simulink model "watertank"  (R2021b)
settings: Solver=FixedStepAuto  StartTime=0.0  StopTime=inf  FixedStep=0.1  RelTol=1e-3
StopFcn:
  | if isLogging
  |     outputJson = jsonencode(struct("simTime", output.simTime, "percentFull", simOutput.percentFull, "pump", simInput.pump, "valve", simInput.valve));
  |     fprintf(outputFile, "%s]", outputJson);
  |     fclose(outputFile);
  | end
model workspace (MAT data in the model file):
  Obj = Simulink.NumericType
  Obj.DataTypeMode = 'Double'
  Obj.SignednessBool = 1
  Obj.WordLength = 64
  Obj.FixedExponent = 0
  Obj.SlopeAdjustmentFactor = 1
  Obj.Bias = 0
  Obj.DataTypeOverride = 'Inherit'
  Obj.IsAlias = 0
  Obj.DataScope = 'Auto'
  PLC_IP_Address = 'localhost'
  pump = 1
  valve = 1
values from neighbouring files (symbols this model uses):
  simInput = struct("pump", 1, "valve", 1)    [initModel.m]
libraries: sh_lib x9, nesl_utility x7, fl_lib x4
PauseFcn:
  | if exist("fixedStepSize", "var") == 0
  |     fixedStepSize = simOutput.SimulationMetadata.ModelInfo.SolverInfo.FixedStepSize;
  | end
  | output.simTime = simOutput.SimulationMetadata.ModelInfo.StopTime - fixedStepSize;
  | output.percentFull = simOutput.percentFull;
ContinueFcn:
  | if isLogging
  |     outputJson = jsonencode(struct("simTime", output.simTime, "percentFull", simOutput.percentFull, "pump", simInput.pump, "valve", simInput.valve));
  |     fprintf(outputFile, "%s,", outputJson);
  | end
settings Model: PacingRate=0.600000  Creator=CCRE  LastModifiedBy=fastsim
settings SolverCC: AlgebraicLoopSolver=TrustRegion
settings DataIOCC: SaveOutput=off  SignalLogging=off  DSMLogging=off  SaveTime=off  ReturnWorkspaceOutputsName=simOutput
settings DebuggingCC: SFMachineParentedDataDiag=warning  ArithmeticOperatorsInVariantConditions=warning
settings SFSimCC: SimUseLocalCustomCode=off  CustomCodeUndefinedFunction=UseInterfaceOnly
settings RTWCC: GenerateReport=on  RTWUseLocalCustomCode=off  BuildConfiguration=Faster Runs  LaunchReport=on
settings CodeAppCC: StateflowObjectComments=on
settings SimscapeCC: SimscapeNormalizeSystem=off

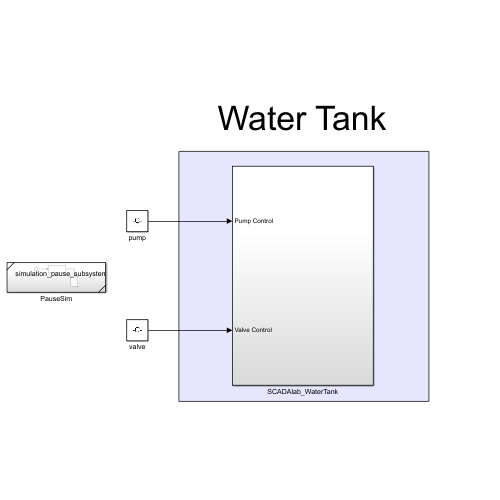
[thumbnail: Simulink's stored preview of the top-level diagram]
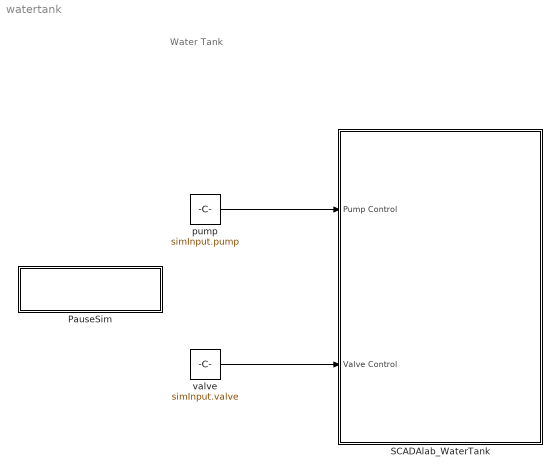
== system watertank ==
  note: Water Tank
  PauseSim : Subsystem  ReferencedSubsystem=simulation_pause_subsystem
  SCADAlab_WaterTank : Subsystem
  pump : Constant  Value=simInput.pump
  valve : Constant  Value=simInput.valve
  wires:
  pump/1 -> SCADAlab_WaterTank/1(Pump Control)
  valve/1 -> SCADAlab_WaterTank/2("Valve Control ")

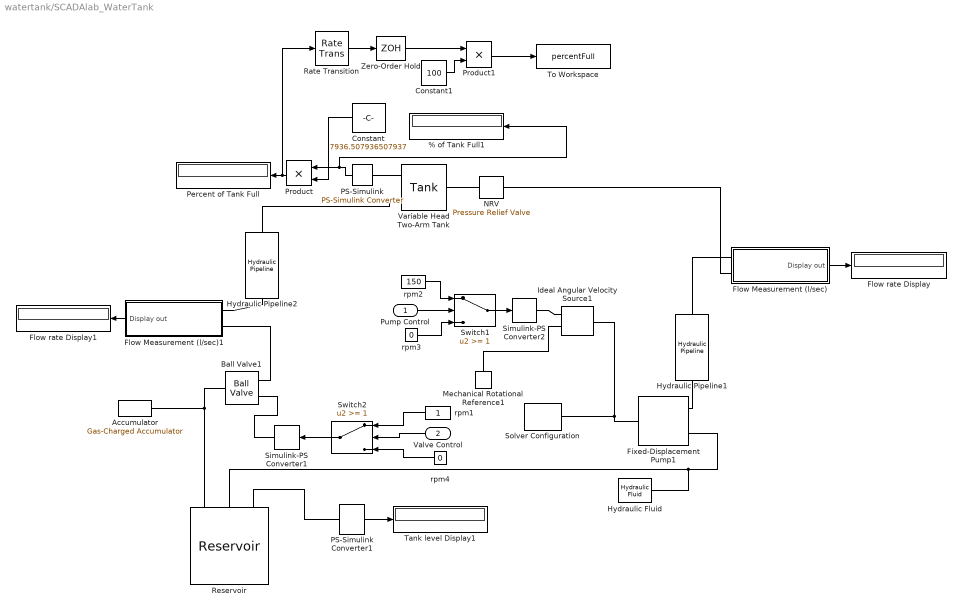
== system watertank/SCADAlab_WaterTank ==
  Pump Control : Inport
  "Valve Control " : Inport  Port=2
  % of Tank Full1 : Display
  Accumulator : sh_lib/Accumulators/Gas-Charged Accumulator  capacity=20 gal  dead_volume=10 gal  pr_preload=0 Pa  k_sh=1.4  stiff_coeff=1e5 Pa/m^3  penetr_coeff=1e5 s*Pa/m^6  flow_rate_specify=off  flow_rate_priority=None  flow_rate=0.005 m^3/s  flow_rate_nominal_specify=off  flow_rate_nominal_unit=m^3/s  flow_rate_nominal_value=1  liquid_volume_specify=on  liquid_volume_priority=High  liquid_volume=0 m^3  liquid_volume_nominal_specify=off  liquid_volume_nominal_unit=m^3  liquid_volume_nominal_value=1  liquid_pressure_specify=off  liquid_pressure_priority=None  liquid_pressure=1.01325e+5 Pa  liquid_pressure_nominal_specify=off  liquid_pressure_nominal_unit=Pa  liquid_pressure_nominal_value=1
      settings: SourceProductBaseCode=SH  InternalSimscapePortConfiguration="{\"Bottom\":[],\"Left\":[],\"Right\":[{\"id\":\"A\",\"label\":\"A\",\"type\":\"foundation.hydraulic.hydraulic\"}],\"Top\":[]}"
  Ball Valve1 : sh_lib/Valves/Flow Control Valves/Ball Valve  valve_seat_spec=1  cone_ang=120 deg  d_ball=3.2 cm  d_orif=3 cm  x_0=0 cm  C_d=0.65  A_leak=1e-12 m^2  lam_spec=2  B_lam=0.999  Re_cr=10  flow_rate_specify=off  flow_rate_priority=None  flow_rate=0.001 m^3/s  flow_rate_nominal_specify=off  flow_rate_nominal_unit=m^3/s  flow_rate_nominal_value=1  pressure_drop_specify=off  pressure_drop_priority=None  pressure_drop=0 Pa  pressure_drop_nominal_specify=off  pressure_drop_nominal_unit=Pa  pressure_drop_nominal_value=1
      settings: SourceProductBaseCode=SH  InternalSimscapePortConfiguration="{\"Bottom\":[],\"Left\":[{\"id\":\"S\",\"label\":\"S\",\"type\":\"input\"},{\"id\":\"A\",\"label\":\"A\",\"type\":\"foundation.hydraulic.hydraulic\"}],\"Right\":[{\"id\":\"B\",\"label\":\"B\",\"type\":\"foundation.hydraulic.hydraulic\"}],\"Top\":[]}"
  Constant : Constant  Value=7936.507936507937
  Constant1 : Constant  Value=100
  Fixed-Displacement Pump1 : sh_lib/Pumps and Motors/Fixed-Displacement Pump  D=0.0271551724137931 l/rev  loss_spec=1  w_nominal=3600 rpm  pr_nominal=.9 bar  visc_nominal=18 cSt  dens_nominal=980 kg/m^3  efficiency_vol=0.92  no_load_torque=0 N*m  torque_pressure_coeff=0.15915*(.0000001)*((0.92)/(0.8)-1 ) N*m/Pa  p_diff_eff_TLU=[100000.0, 1000000.0, 2000000.0] Pa  omega_eff_TLU=[25.0, 50.0, 100.0, 200.0, 300.0, 400.0] rad/s  vol_eff_TLU=[0.816, 0.908, 0.954, 0.977, 0.981, 0.984; 0.325, 0.663, 0.831, 0.916, 0.925, 0.946; 0.137, 0.568, 0.78, 0.892, 0.893, 0.91]  mech_eff_TLU=[0.996, 0.996, 0.996, 0.996, 0.996, 0.996; 0.988, 0.989, 0.989, 0.989, 0.989, 0.99; 0.981, 0.981, 0.982, 0.982, 0.983, 0.984]  p_diff_loss_TLU=[100000.0, 1000000.0, 2000000.0] Pa  omega_loss_TLU=[25.0, 50.0, 100.0, 200.0, 300.0, 400.0] rad/s  vol_loss_TLU=[0.023, 0.023, 0.023, 0.023, 0.0285, 0.032; 0.0844, 0.0842, 0.0845, 0.084, 0.1125, 0.108; 0.1079, 0.108, 0.11, 0.108, 0.1605, 0.18] * 1e-3 m^3/s  mech_loss_TLU=[0.002, 0.002, 0.002, 0.002, 0.002, 0.002; 0.0607, 0.0556, 0.0556, 0.0556, 0.0556, 0.0505; 0.1937, 0.1937, 0.1833, 0.1833, 0.1729, 0.1626] N*m  pressure_threshold=1e5 Pa  omega_threshold=10 rad/s  quadrant_check=0  pressure_check=0  min_valid_pressure=0 Pa  vol_eff_min=1e-3  vol_eff_max=1  mech_eff_min=1e-3  mech_eff_max=1
      settings: SourceProductBaseCode=SH  InternalSimscapePortConfiguration="{\"Bottom\":[],\"Left\":[{\"id\":\"S\",\"label\":\"S\",\"type\":\"foundation.mechanical.rotational.rotational\"}],\"Right\":[{\"id\":\"P\",\"label\":\"P\",\"type\":\"foundation.hydraulic.hydraulic\"},{\"id\":\"T\",\"label\":\"T\",\"type\":\"foundation.hydraulic.hydraulic\"}],\"Top\":[]}"
  Flow Measurement (l/sec) : Subsystem
  Flow Measurement (l/sec)1 : Subsystem
  Flow rate Display : Display
  Flow rate Display1 : Display
  Hydraulic Fluid : sh_lib/Hydraulic Utilities/Hydraulic Fluid  DataSource=1  SelFluid=24  SysTemp=30  TrapAir=0.005  ViscDerFactor=1  range_error=1
  Hydraulic Pipeline1 : sh_lib/Pipelines/Hydraulic Pipeline  cs_type=1  d_in=.5 cm  area=1e-4 m^2  D_h=0.0112 m  s_factor=64  length=140 cm  length_ad=140 cm  roughness=1.5e-2 cm  Re_lam=2e+3  Re_turb=4e+3  wall_type=1  pr_r_coef=2e-12 m/Pa  time_const=0.01 s  k_sh=1.4  initial_pressure=0 Pa
      settings: SourceProductBaseCode=SH  InternalSimscapePortConfiguration="{\"Bottom\":[],\"Left\":[{\"id\":\"A\",\"label\":\"A\",\"type\":\"foundation.hydraulic.hydraulic\"}],\"Right\":[{\"id\":\"B\",\"label\":\"B\",\"type\":\"foundation.hydraulic.hydraulic\"}],\"Top\":[]}"
  Hydraulic Pipeline2 : sh_lib/Pipelines/Hydraulic Pipeline  cs_type=1  d_in=.7 cm  area=1e-4 m^2  D_h=0.0112 m  s_factor=64  length=90 cm  length_ad=10 cm  roughness=1.5e-3 cm  Re_lam=2e+3  Re_turb=4e+3  wall_type=1  pr_r_coef=2e-12 m/Pa  time_const=0.01 s  k_sh=1.4  initial_pressure=0 Pa
      settings: SourceProductBaseCode=SH  InternalSimscapePortConfiguration="{\"Bottom\":[],\"Left\":[{\"id\":\"A\",\"label\":\"A\",\"type\":\"foundation.hydraulic.hydraulic\"}],\"Right\":[{\"id\":\"B\",\"label\":\"B\",\"type\":\"foundation.hydraulic.hydraulic\"}],\"Top\":[]}"
  Ideal Angular Velocity Source1 : fl_lib/Mechanical/Mechanical Sources/Ideal Angular Velocity Source
  Mechanical Rotational Reference1 : fl_lib/Mechanical/Rotational Elements/Mechanical Rotational Reference
  NRV : sh_lib/Valves/Pressure Control Valves/Pressure Relief Valve  valve_area_spec=1  p_diff_TLU=[30.15e5 : 15e3 : 31.35e5] Pa  area_TLU=[1 : 1 : 9] .* 1e-5 m^2  area_max=1e-4 m^2  pres_set=0.001 Pa  reg_range=5e5 Pa  C_d=0.7  A_leak=1e-12 m^2  lam_spec=2  B_lam=0.999  Re_cr=12  dynamic=0  tau=0.1 s  area_init=1e-12 m^2
      settings: SourceProductBaseCode=SH  InternalSimscapePortConfiguration="{\"Bottom\":[],\"Left\":[{\"id\":\"A\",\"label\":\"A\",\"type\":\"foundation.hydraulic.hydraulic\"}],\"Right\":[{\"id\":\"B\",\"label\":\"B\",\"type\":\"foundation.hydraulic.hydraulic\"}],\"Top\":[]}"
  "PS-Simulink " : nesl_utility/PS-Simulink Converter  PhysicalDomain=network_engine_domain  SubClassName=ps_output  LeftPortType=input  RightPortType=output  PseudoPeriodic=off  Frequencies=[]  Unit=1  AffineConversion=off
      settings: SourceProductBaseCode=PW,SS
  PS-Simulink Converter1 : nesl_utility/PS-Simulink Converter  PhysicalDomain=network_engine_domain  SubClassName=ps_output  LeftPortType=input  RightPortType=output  PseudoPeriodic=off  Frequencies=[]  Unit=1  AffineConversion=off
      settings: SourceProductBaseCode=PW,SS
  Percent of Tank Full : Display
  Product : Product
  Product1 : Product
  Rate Transition : RateTransition
  Reservoir : sh_lib/Hydraulic Utilities/Reservoir  press=0 Pa  init_volume=1000000 l  ret_diam=.5 cm  loss_coeff=1
      settings: SourceProductBaseCode=SH  InternalSimscapePortConfiguration="{\"Bottom\":[],\"Left\":[{\"id\":\"V\",\"label\":\"V\",\"type\":\"output\"},{\"id\":\"P\",\"label\":\"P\",\"type\":\"foundation.hydraulic.hydraulic\"},{\"id\":\"R\",\"label\":\"R\",\"type\":\"foundation.hydraulic.hydraulic\"}],\"Right\":[],\"Top\":[]}"
  Simulink-PS Converter1 : nesl_utility/Simulink-PS Converter  PhysicalDomain=network_engine_domain  SubClassName=ps_input  LeftPortType=input  RightPortType=output  PseudoPeriodic=off  Frequencies=[]  NoiseDistribution=none  NoiseParameters=[]  Unit=1  AffineConversion=off  FilteringAndDerivatives=zero  SimscapeFilterOrder=1  InputFilterTimeConstant=0.001  UdotUserProvided=1
      settings: SourceProductBaseCode=PW,SS
  Simulink-PS Converter2 : nesl_utility/Simulink-PS Converter  PhysicalDomain=network_engine_domain  SubClassName=ps_input  LeftPortType=input  RightPortType=output  PseudoPeriodic=off  Frequencies=[]  NoiseDistribution=none  NoiseParameters=[]  Unit=1  AffineConversion=off  FilteringAndDerivatives=zero  SimscapeFilterOrder=1  InputFilterTimeConstant=0.001  UdotUserProvided=1
      settings: SourceProductBaseCode=PW,SS
  Solver Configuration : nesl_utility/Solver Configuration  PhysicalDomain=network_engine_domain  SubClassName=solver  LeftPortType=input  RightPortType=generic  Tones=[]  Harmonics=[]  SimulateNoise=off  Profile=off  UseLocalSampling=off  EnableSwitchedLinearOptims=on  FrequencyDomain=off  UseCCode=off  RelTol=0.001  AbsTol=1e-06  MinStep=1e-09  ToWorkspace=off  RevertToSquareIcSolve=off  NumHomotopyIterations=100  PhasorMode=off  PhasorModeNumHarmonics=1  DoDC=off  ResidualTolerance=1  UseLocalSolver=on  LocalSolverChoice=NE_TRAPEZOIDAL_ADVANCER  LocalSolverSampleTime=0.1  DoFixedCost=on  MaxNonlinIter=12  MaxModeIter=2  ComputeImpulses=off  ImpulseIterations=2  LinearAlgebra=Full  EquationFormulation=NE_TIME_EF  DelaysMemoryBudget=1024  AutomaticFiltering=on  FilteringTimeConstant=0.001  PartitionStorageMethod=AS_NEEDED  PartitionMemoryBudget=1024  PartitionMethod=FAST
      settings: SourceProductBaseCode=PW,SS
  Switch1 : Switch  Threshold=1
  Switch2 : Switch  Threshold=1
  Tank level Display1 : Display
  To Workspace : ToWorkspace  VariableName=percentFull  SampleTime=-1
      settings: MaxDataPoints=1  Save2DSignal=2-D array (concatenate along first dimension)
  Variable Head Two-Arm Tank : sh_lib/Low-Pressure Blocks/Tank  press=0 Pa  level_spec=1  tank_area=.0314 m^2  fluid_volume_tab=[ 0 0.0028 0.0065 0.0114 0.0176 0.0252 0.0344 0.0436 0.0512 0.0574 0.0623 0.066 0.0688 0.0707 0.07199999999999999 0.0727 ] m^3  fluid_level_tab=[ 0 0.02 0.04 0.06 0.08 0.1 0.12 0.14 0.16 0.18 0.2 0.22 0.24 0.26 0.28 0.3 ] m  interp_method=1  extrap_method=1  pipe_diam=0.02 m  loss_coeff=1.2  g=9.80665 m/s^2  min_level=1e-3 m  fluid_level_check=0  volume_specify=on  volume_priority=High  volume=0 l  volume_nominal_specify=off  volume_nominal_unit=l  volume_nominal_value=1  level_specify=off  level_priority=None  level=0.025 m  level_nominal_specify=off  level_nominal_unit=m  level_nominal_value=1  pipe_diam_A=0.2 m  loss_coeff_A=1.2  height_B=38 cm  pipe_diam_B=0.2 m  loss_coeff_B=1.2  height_C=0.8 m  pipe_diam_C=0.02 m  loss_coeff_C=1.2
      settings: SourceProductBaseCode=SH  InternalSimscapePortConfiguration="{\"Bottom\":[],\"Left\":[{\"id\":\"B\",\"label\":\"B\",\"type\":\"foundation.hydraulic.hydraulic\"}],\"Right\":[{\"id\":\"V\",\"label\":\"V\",\"type\":\"output\"},{\"id\":\"A\",\"label\":\"A\",\"type\":\"foundation.hydraulic.hydraulic\"}],\"Top\":[]}"
  Zero-Order Hold : ZeroOrderHold  SampleTime=0.1
  rpm1 : Constant
  rpm2 : Constant  Value=150
  rpm3 : Constant  Value=0
  rpm4 : Constant  Value=0
  wires:
  Flow Measurement (l/sec)1/1(Display out) -> Flow rate Display1/1
  PS-Simulink Converter1/1 -> Tank level Display1/1
  Flow Measurement (l/sec)/1(Display out) -> Flow rate Display/1
  Constant/1 -> Product/2
  "PS-Simulink "/1 -> % of Tank Full1/1, Product/1
  rpm3/1 -> Switch1/3
  rpm2/1 -> Switch1/1
  Pump Control/1 -> Switch1/2
  Switch1/1 -> Simulink-PS Converter2/1
  rpm4/1 -> Switch2/3
  rpm1/1 -> Switch2/1
  Switch2/1 -> Simulink-PS Converter1/1
  "Valve Control "/1 -> Switch2/2
  Product/1 -> Rate Transition/1, Percent of Tank Full/1
  Rate Transition/1 -> Zero-Order Hold/1
  Constant1/1 -> Product1/2
  Zero-Order Hold/1 -> Product1/1
  Product1/1 -> To Workspace/1
  connections:
  Variable Head Two-Arm Tank/LConn1 -- NRV/RConn1
  Hydraulic Pipeline1/LConn1 -- Flow Measurement (l/sec)/LConn1
  Variable Head Two-Arm Tank/RConn1 -- "PS-Simulink "/LConn1
  Solver Configuration/RConn1 -- Ideal Angular Velocity Source1/LConn1 -- Fixed-Displacement Pump1/LConn1
  Mechanical Rotational Reference1/LConn1 -- Ideal Angular Velocity Source1/RConn2
  Reservoir/LConn2 -- Fixed-Displacement Pump1/RConn2 -- Hydraulic Fluid/RConn1
  Simulink-PS Converter2/RConn1 -- Ideal Angular Velocity Source1/RConn1
  PS-Simulink Converter1/LConn1 -- Reservoir/LConn1
  NRV/LConn1 -- Flow Measurement (l/sec)/LConn2
  Hydraulic Pipeline1/RConn1 -- Fixed-Displacement Pump1/RConn1
  Simulink-PS Converter1/RConn1 -- Ball Valve1/LConn1
  Reservoir/LConn3 -- Ball Valve1/RConn1 -- Accumulator/RConn1
  Flow Measurement (l/sec)1/LConn2 -- Ball Valve1/LConn2
  Flow Measurement (l/sec)1/LConn1 -- Hydraulic Pipeline2/RConn1
  Variable Head Two-Arm Tank/RConn2 -- Hydraulic Pipeline2/LConn1

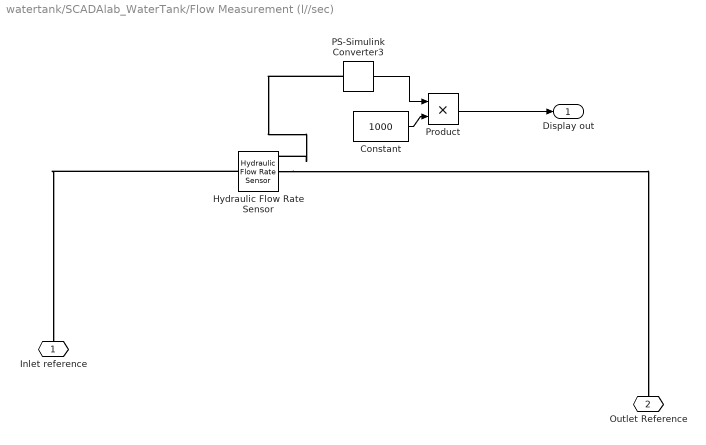
== system watertank/SCADAlab_WaterTank/Flow Measurement (l//sec) ==
  Constant : Constant  Value=1000
  Hydraulic Flow Rate Sensor : fl_lib/Hydraulic/Hydraulic Sensors/Hydraulic Flow Rate Sensor
  PS-Simulink Converter3 : nesl_utility/PS-Simulink Converter  PhysicalDomain=network_engine_domain  SubClassName=ps_output  LeftPortType=input  RightPortType=output  PseudoPeriodic=off  Frequencies=[]  Unit=m^3/s  AffineConversion=off
      settings: SourceProductBaseCode=PW,SS
  Product : Product
  Inlet reference : PMIOPort  Side=Left
  " Outlet Reference" : PMIOPort  Port=2  Side=Left
  Display out : Outport
  wires:
  Product/1 -> Display out/1
  Constant/1 -> Product/2
  PS-Simulink Converter3/1 -> Product/1
  connections:
  PS-Simulink Converter3/LConn1 -- Hydraulic Flow Rate Sensor/RConn1
  Hydraulic Flow Rate Sensor/RConn2 -- " Outlet Reference"/RConn1
  Hydraulic Flow Rate Sensor/LConn1 -- Inlet reference/RConn1

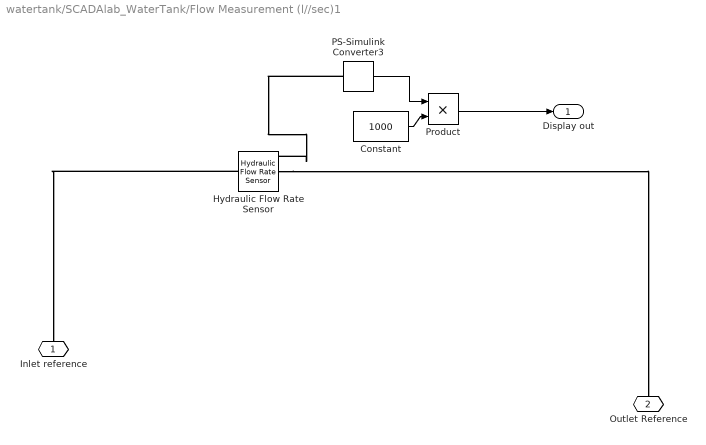
== system watertank/SCADAlab_WaterTank/Flow Measurement (l//sec)1 ==
  Constant : Constant  Value=1000
  Hydraulic Flow Rate Sensor : fl_lib/Hydraulic/Hydraulic Sensors/Hydraulic Flow Rate Sensor
  PS-Simulink Converter3 : nesl_utility/PS-Simulink Converter  PhysicalDomain=network_engine_domain  SubClassName=ps_output  LeftPortType=input  RightPortType=output  PseudoPeriodic=off  Frequencies=[]  Unit=m^3/s  AffineConversion=off
      settings: SourceProductBaseCode=PW,SS
  Product : Product
  Inlet reference : PMIOPort  Side=Left
  " Outlet Reference" : PMIOPort  Port=2  Side=Left
  Display out : Outport
  wires:
  Product/1 -> Display out/1
  Constant/1 -> Product/2
  PS-Simulink Converter3/1 -> Product/1
  connections:
  PS-Simulink Converter3/LConn1 -- Hydraulic Flow Rate Sensor/RConn1
  Hydraulic Flow Rate Sensor/RConn2 -- " Outlet Reference"/RConn1
  Hydraulic Flow Rate Sensor/LConn1 -- Inlet reference/RConn1
